simulink model "interp_compare_2d_lut_R2019a"  (R2019a)
settings: Solver=FixedStepDiscrete  StartTime=0.0  StopTime=1  FixedStep=1  RelTol=1e-3
Description:
  | 2-D Lookup Table: Lagrange vs point-slope
settings Model: Creator=Administrator  LastModifiedBy=Administrator
settings DebuggingCC: UnconnectedInputMsg=none  UnconnectedOutputMsg=none  UnconnectedLineMsg=none
settings ModelReferenceCC: UpdateModelReferenceTargets=IfOutOfDate  EnableRefExpFcnMdlSchedulingChecks=off
settings RTWCC: Description=Generic Real-Time Target
settings ConfigComp: CovBoundaryAbsTol=1.0e-5

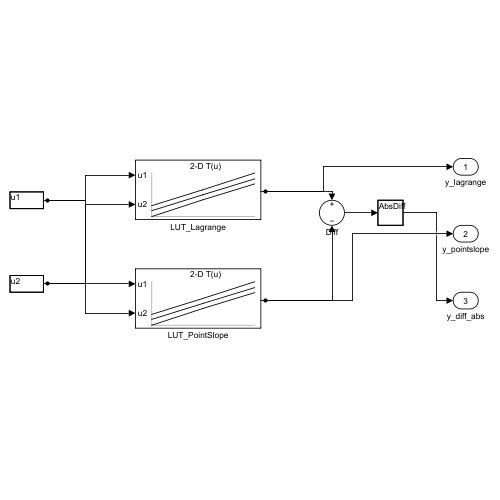
[thumbnail: Simulink's stored preview of the top-level diagram]
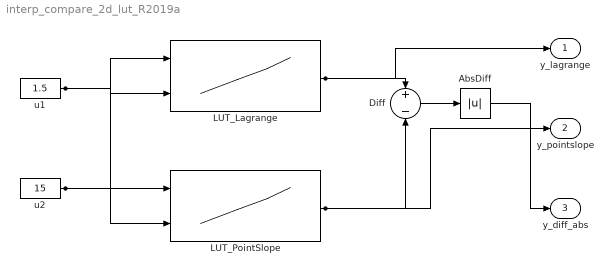
== system interp_compare_2d_lut_R2019a ==
  AbsDiff : Abs
  Diff : Sum  Inputs=+-
  LUT_Lagrange : Lookup_n-D  BreakpointsForDimension1=[1 2 3]  BreakpointsForDimension2=[10 20 30]  Table=[100 200 300;400 500 600;700 800 900]  InterpMethod=Linear Lagrange  ExtrapMethod=Clip  InternalRulePriority=Speed  RndMeth=Simplest  InputSameDT=on
  LUT_PointSlope : Lookup_n-D  BreakpointsForDimension1=[1 2 3]  BreakpointsForDimension2=[10 20 30]  Table=[100 200 300;400 500 600;700 800 900]  ExtrapMethod=Clip  InternalRulePriority=Speed  RndMeth=Simplest  InputSameDT=on
  u1 : Constant  Value=1.5
  u2 : Constant  Value=15
  y_lagrange : Outport
  y_pointslope : Outport  Port=2
  y_diff_abs : Outport  Port=3
  wires:
  u1/1 -> LUT_Lagrange/1, LUT_PointSlope/1
  u2/1 -> LUT_Lagrange/2, LUT_PointSlope/2
  LUT_Lagrange/1 -> Diff/1, y_lagrange/1
  LUT_PointSlope/1 -> Diff/2, y_pointslope/1
  Diff/1 -> AbsDiff/1
  AbsDiff/1 -> y_diff_abs/1
